simulink model "hinf_747c"  (Simulink 7.8)
settings: Solver=ode45  StartTime=0.0  StopTime=10.0  RelTol=1e-3
undefined symbols (not defined in the file): a, b, c, d, K2
settings Model: Creator=Dan  LastModifiedBy=Dan
settings DebuggingCC: InitInArrayFormatMsg=none

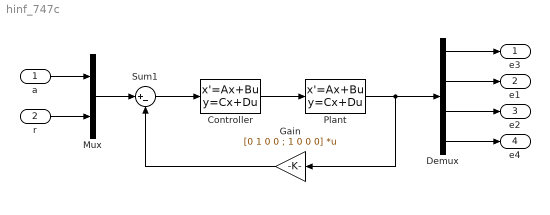
== system hinf_747c ==
  a : Inport
  r : Inport  Port=2
  Controller : StateSpace  A=K2.A  B=K2.B  C=K2.C  D=K2.D
  Demux : Demux
  Gain : Gain  Gain=[0 1 0 0 ; 1 0 0 0]  Multiplication=Matrix(K*u)
  Mux : Mux  Inputs=2
  Plant : StateSpace  A=a  B=b  C=c  D=d
  Sum1 : Sum  Inputs=|+-
  e3 : Outport
  e1 : Outport  Port=2
  e2 : Outport  Port=3
  e4 : Outport  Port=4
  wires:
  Plant/1 -> Gain/1, Demux/1
  Sum1/1 -> Controller/1
  Controller/1 -> Plant/1
  Gain/1 -> Sum1/2
  Mux/1 -> Sum1/1
  a/1 -> Mux/1
  r/1 -> Mux/2
  Demux/1 -> e3/1
  Demux/2 -> e1/1
  Demux/3 -> e2/1
  Demux/4 -> e4/1
